simulink model "suspensao_passiva"  (R2025a)
settings: Solver=VariableStepAuto  StartTime=0.0  StopTime=t_sim  RelTol=1e-3
undefined symbols (not defined in the file): c_passivo, duracao_lombada, h_lombada, k_s, k_t, m_s, m_us, t_inicio_lombada, t_sim
settings Model: Creator=Anderson  LastModifiedBy=Anderson

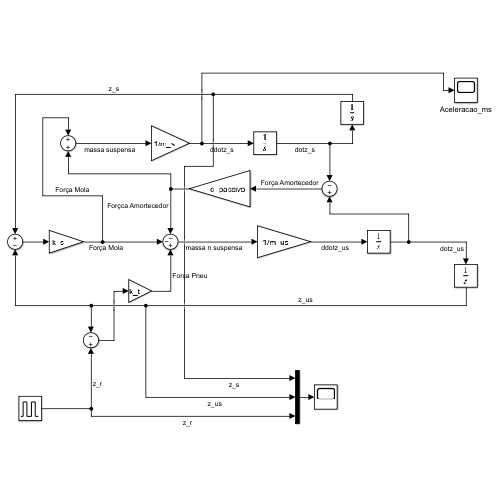
[thumbnail: Simulink's stored preview of the top-level diagram]
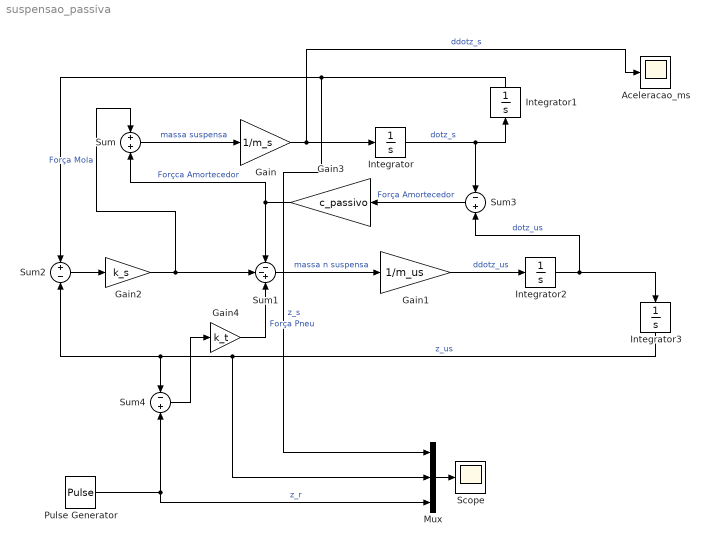
== system suspensao_passiva ==
  Aceleracao_ms : Scope
  Gain : Gain  Gain=1/m_s
  Gain1 : Gain  Gain=1/m_us
  Gain2 : Gain  Gain=k_s
  Gain3 : Gain  Gain=c_passivo
  Gain4 : Gain  Gain=k_t
  Integrator{,1..3} (4 alike) : Integrator
  Mux : Mux  Inputs=3
  Pulse Generator : DiscretePulseGenerator  PulseType=Time based  Amplitude=h_lombada  Period=t_sim  PulseWidth=(duracao_lombada/t_sim)*100  PhaseDelay=t_inicio_lombada
  Scope : Scope
  Sum : Sum
  Sum1 : Sum  Inputs=--+
  Sum2 : Sum  Inputs=+-
  Sum3 : Sum  Inputs=-+
  Sum4 : Sum  Inputs=-+
  wires:
  Sum/1 -> Gain/1  "massa suspensa"
  Gain/1 -> Aceleracao_ms/1, Integrator/1  "ddotz_s"
  Integrator/1 -> Integrator1/1, Sum3/1  "dotz_s"
  Integrator1/1 -> Mux/1, Sum2/1  "z_s"
  Sum3/1 -> Gain3/1  "Força Amortecedor"
  Gain2/1 -> Sum/1, Sum1/2  "Força Mola"
  Gain4/1 -> Sum1/3  "Força Pneu"
  Sum1/1 -> Gain1/1  "massa n suspensa"
  Gain1/1 -> Integrator2/1  "ddotz_us"
  Integrator2/1 -> Integrator3/1, Sum3/2  "dotz_us"
  Integrator3/1 -> Mux/2, Sum4/1, Sum2/2  "z_us"
  Sum2/1 -> Gain2/1
  Gain3/1 -> Sum/2, Sum1/1  "Forçca Amortecedor"
  Pulse Generator/1 -> Sum4/2, Mux/3  "z_r"
  Sum4/1 -> Gain4/1
  Mux/1 -> Scope/1
